simulink model "Written_SS_V_S_Input_LongV_LatV_Yaw_Output"  (R2018b)
settings: Solver=VariableStepAuto  StartTime=0.0  StopTime=10.0  RelTol=1e-3
undefined symbols (not defined in the file): Cf, Cr, Iz, lf, lr, m
settings Model: Creator=Johan PC  LastModifiedBy=Johan PC

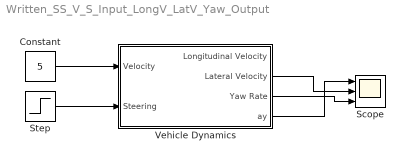
== system Written_SS_V_S_Input_LongV_LatV_Yaw_Output ==
  Constant : Constant  Value=5
  Scope : Scope  NumInputPorts=3
  Step : Step  Time=0.3  After=0.1  SampleTime=0
  Vehicle Dynamics : Subsystem
  wires:
  Constant/1 -> Vehicle Dynamics/1(Velocity)
  Step/1 -> Vehicle Dynamics/2(Steering)
  Vehicle Dynamics/2(Lateral Velocity) -> Scope/2
  Vehicle Dynamics/3(Yaw Rate) -> Scope/3
  Vehicle Dynamics/4(ay) -> Scope/1

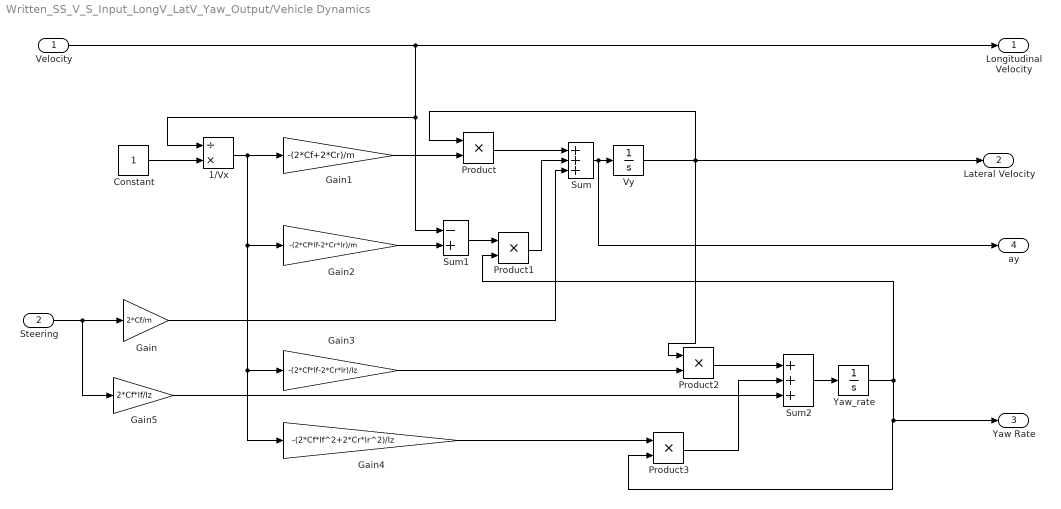
== system Written_SS_V_S_Input_LongV_LatV_Yaw_Output/Vehicle Dynamics ==
  Velocity : Inport
  Steering : Inport  Port=2
  1/Vx : Product  Inputs=/*
  Constant : Constant
  Gain : Gain  Gain=2*Cf/m
  Gain1 : Gain  Gain=-(2*Cf+2*Cr)/m
  Gain2 : Gain  Gain=-(2*Cf*lf-2*Cr*lr)/m
  Gain3 : Gain  Gain=-(2*Cf*lf-2*Cr*lr)/Iz
  Gain4 : Gain  Gain=-(2*Cf*lf^2+2*Cr*lr^2)/Iz
  Gain5 : Gain  Gain=2*Cf*lf/Iz
  Product{,1..3} (4 alike) : Product
  Sum : Sum  Inputs=+++
  Sum1 : Sum  Inputs=-+
  Sum2 : Sum  Inputs=+++
  Vy : Integrator
  "Yaw_rate " : Integrator
  Longitudinal Velocity : Outport
  Lateral Velocity : Outport  Port=2
  Yaw Rate : Outport  Port=3
  ay : Outport  Port=4
  wires:
  Sum2/1 -> "Yaw_rate "/1
  Gain2/1 -> Sum1/2
  Gain4/1 -> Product3/1
  Constant/1 -> 1/Vx/2
  Gain3/1 -> Product2/2
  1/Vx/1 -> Gain4/1, Gain3/1, Gain2/1, Gain1/1
  Product2/1 -> Sum2/1
  Product3/1 -> Sum2/2
  Gain5/1 -> Sum2/3
  Sum1/1 -> Product1/1
  "Yaw_rate "/1 -> Yaw Rate/1, Product3/2, Product1/2
  Gain/1 -> Sum/3
  Steering/1 -> Gain/1, Gain5/1
  Gain1/1 -> Product/2
  Product/1 -> Sum/1
  Vy/1 -> Product2/1, Product/1, Lateral Velocity/1
  Sum/1 -> ay/1, Vy/1
  Velocity/1 -> Longitudinal Velocity/1, 1/Vx/1, Sum1/1
  Product1/1 -> Sum/2
